simulink model "fm_maja"  (R2025b)
settings: Solver=ode2  StartTime=0.0  StopTime=5  FixedStep=vehicle.sampletime  RelTol=1e-3  EnableMultiTasking=on
undefined symbols (not defined in the file or in its folder): battery, constants, Earth, engine, F, Light, MIL, propeller, servo, vehicle, WGS84
libraries: sharedtransform x3, aerolibwind2 x2, aerolibutil x2, aerolib6dof2 x1, aerolibatmos2 x1, aerolibtransform2 x1, simulink x1, aerolibobsolete x1
settings Model: Creator=ac112430  LastModifiedBy=ac124458
settings SolverCC: AlgebraicLoopSolver=TrustRegion
settings DataIOCC: ReturnWorkspaceOutputs=off
settings OptimizationCC: ReuseModelBlockBuffer=off  LifeSpan=inf
settings DebuggingCC: UnconnectedInputMsg=warning  UnconnectedOutputMsg=warning  UnconnectedLineMsg=warning  SFUnexpectedBacktrackingDiag=warning  SFNoUnconditionalDefaultTransitionDiag=warning  SFExecutionAtInitializationDiag=none  ArithmeticOperatorsInVariantConditions=warning
settings ModelReferenceCC: EnableRefExpFcnMdlSchedulingChecks=on
settings SFSimCC: SimUseLocalCustomCode=off  CustomCodeUndefinedFunction=UseInterfaceOnly
settings RTWCC: RTWUseLocalCustomCode=off  GPUComputeCapability=3.5
settings CodeAppCC: StateflowObjectComments=on
settings GRTTargetCC: TargetLangStandard=C89/C90 (ANSI)
settings ConfigComp: CovMetricSettings=dw  CovSaveCumulativeToWorkspaceVar=on  CovSaveSingleToWorkspaceVar=on  CovExternalEMLEnable=off

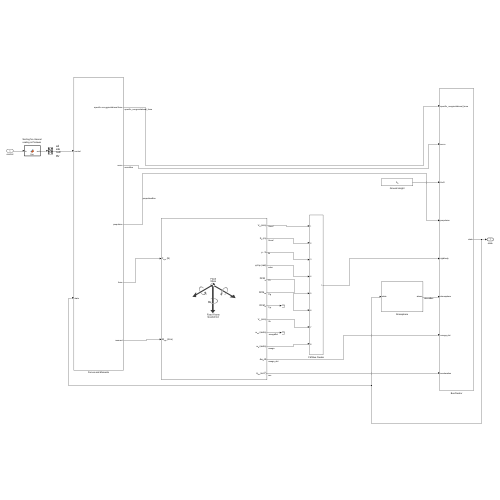
[thumbnail: Simulink's stored preview of the top-level diagram]
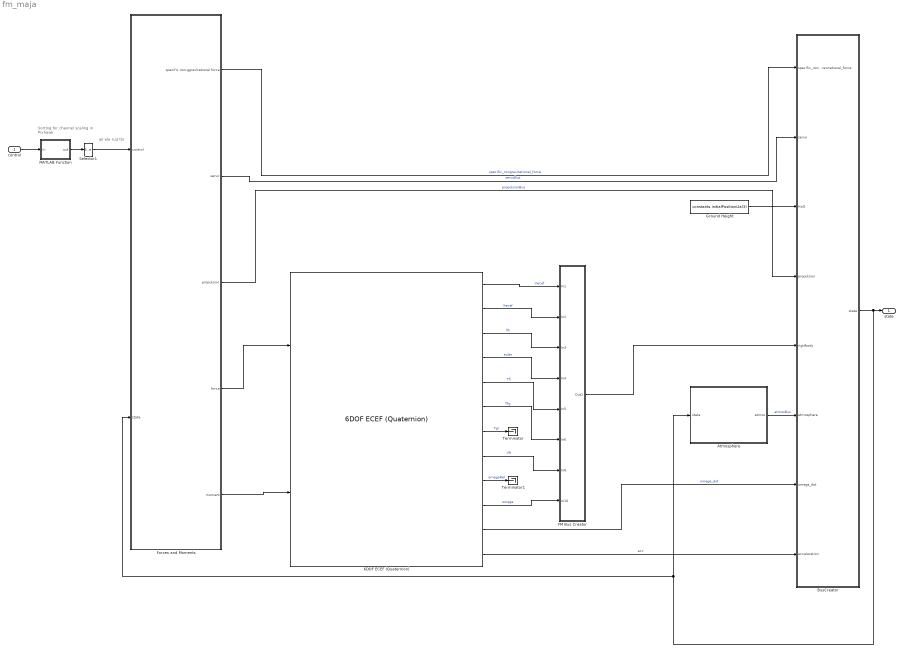
== system fm_maja ==
  note: ail
      | ele
      | rud
      | thr
  note: Sorting for channel
      | scaling in Pixhawk
  control : Inport  PortDimensions=4
  6DOF ECEF (Quaternion) : aerolib6dof2/6DOF ECEF (Quaternion)  units=Metric (MKS)  mtype=Fixed  xg_0=vehicle.pos0  Vm_0=vehicle.v0  eul_0=vehicle.ori0  pm_0=vehicle.omega0  mass_0=vehicle.m  mass_e=0.5  mass_f=2.0  inertia=vehicle.J  inertia_e=eye(3)  inertia_f=2*eye(3)  vre_flag=on  abi_flag=off  ptype=Earth (WGS84)  R=6378137  F=1/298.257223563  w_E=7292115e-11  angle_in=Internal  LPM0=0  quat_statename=''  pm_statename=''  Vm_statename=''  posfixedframe_statename=''  posinertial_statename=''  LPM_statename=''  mass_statename=''
  Atmosphere : Subsystem
  BusCreator : Subsystem
  FM Bus Creator : Subsystem
  Forces and Moments : Subsystem
  Ground Height : Constant  Value=constants.initialPositionLla(3)  SampleTime=-1
      mask Display: disp('h_0', 'texmode', 'on');
  MATLAB Function : MATLAB Function  TreatAsAtomicUnit=on
  Selector1 : Selector  InputPortWidth=4  IndexOptions=Index vector (dialog)  Indices=[2 3 4 1]  OutputSizes=1  RuntimeRangeChecks=on
  Terminator : Terminator
  Terminator1 : Terminator
  state : Outport  OutDataTypeStr=Bus: fmBus  VectorParamsAs1DForOutWhenUnconnected=off
  wires:
  6DOF ECEF (Quaternion)/11 -> BusCreator/7(omega_dot)  "omega_dot"
  BusCreator/1(state) -> Atmosphere/1(state), Forces and Moments/2(state), state/1
  Atmosphere/1(atmos) -> BusCreator/6(atmosphere)  "atmosBus"
  Forces and Moments/1(specific non-ggravitational force) -> BusCreator/1(specific_nongravitational_force)  "specific_nongravitational_force"
  Forces and Moments/2(servo) -> BusCreator/2(servo)  "servoBus"
  Forces and Moments/3(propulsion) -> BusCreator/4(propulsion)  "propulsionBus"
  Forces and Moments/5(moment) -> 6DOF ECEF (Quaternion)/2
  Forces and Moments/4(force) -> 6DOF ECEF (Quaternion)/1
  control/1 -> MATLAB Function/1(in)
  Ground Height/1 -> BusCreator/3(HoG)
  6DOF ECEF (Quaternion)/12 -> BusCreator/8(acceleration)  "acc"
  6DOF ECEF (Quaternion)/1 -> FM Bus Creator/1(In1)  "Vecef"
  6DOF ECEF (Quaternion)/2 -> FM Bus Creator/2(In2)  "Xecef"
  6DOF ECEF (Quaternion)/3 -> FM Bus Creator/3(In3)  "llh"
  6DOF ECEF (Quaternion)/4 -> FM Bus Creator/4(In4)  "euler"
  6DOF ECEF (Quaternion)/5 -> FM Bus Creator/5(In5)  "Tfi"
  6DOF ECEF (Quaternion)/6 -> FM Bus Creator/6(In6)  "Tfg"
  6DOF ECEF (Quaternion)/8 -> FM Bus Creator/7(In8)  "Vb"
  6DOF ECEF (Quaternion)/10 -> FM Bus Creator/8(In10)  "omega"
  FM Bus Creator/1(Out1) -> BusCreator/5(rigidbody)
  6DOF ECEF (Quaternion)/9 -> Terminator1/1  "omegaRel"
  6DOF ECEF (Quaternion)/7 -> Terminator/1  "Tgr"
  MATLAB Function/1(out) -> Selector1/1
  Selector1/1 -> Forces and Moments/1(control)

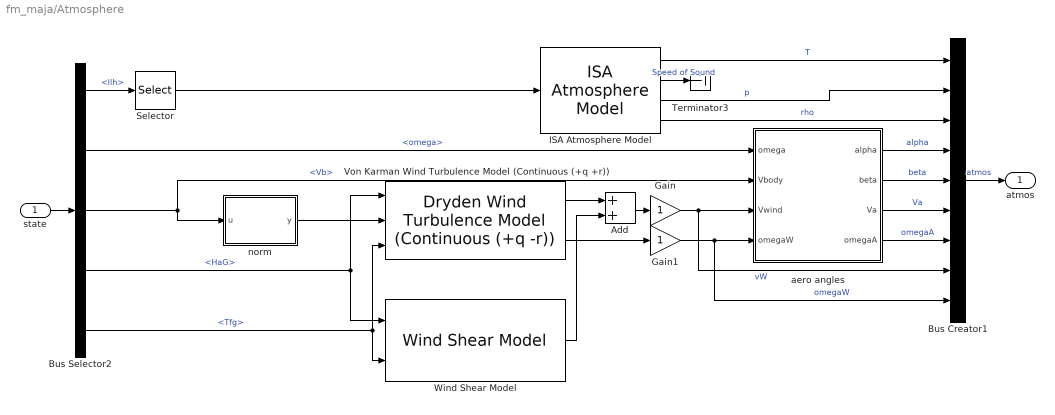
== system fm_maja/Atmosphere ==
  state : Inport
  Add : Sum
  Bus Creator1 : BusCreator  Inputs=9  OutDataTypeStr=Bus: atmosBus
  Bus Selector2 : BusSelector  OutputSignals=rigidbodyBus.llh,rigidbodyBus.omega,rigidbodyBus.Vb,utilityBus.HaG,rigidbodyBus.Tfg
  Gain : Gain
  Gain1 : Gain
  ISA Atmosphere Model : aerolibatmos2/ISA Atmosphere Model  useExtended=off  action=Warning  custom=off  viscosityOut=off  g=9.80665  gamma=1.4  R=287.0531  L=0.0065  h_trop=11000  h_strat=20000  rho0=1.225  P0=101325  T0=288.15  h0=0  S=110.4  Tref=273.15  muref=1.716e-5
  Selector : Selector  InputPortWidth=3  IndexOptions=Index vector (dialog)  Indices=3  OutputSizes=1
  Terminator3 : Terminator
  Von Karman Wind Turbulence Model (Continuous (+q +r)) : aerolibwind2/Dryden Wind Turbulence Model  (Continuous (+q -r))  units=Metric (MKS)  spec=MIL-F-8785C  model=Continuous Von Karman (+q +r)  W20=atmosphere.windStrength  Wdeg=atmosphere.windDir  TurbProb=10^-2 - Light  L_high=410  Wingspan=aerodynamic.b  ts=vehicle.sampletime  Seed=randi(20000,1,4)  T_on=off
  Wind Shear Model : aerolibwind2/Wind Shear Model  units=Metric (MKS)  phase=Other  W_20=atmosphere.windStrength  Wdeg=atmosphere.windDir
  aero angles : MATLAB Function  TreatAsAtomicUnit=on
  norm : MATLAB Function  TreatAsAtomicUnit=on
  atmos : Outport  VectorParamsAs1DForOutWhenUnconnected=off
  wires:
  Bus Creator1/1 -> atmos/1  "atmos"
  ISA Atmosphere Model/3 -> Bus Creator1/2  "p"
  ISA Atmosphere Model/1 -> Bus Creator1/1  "T"
  ISA Atmosphere Model/2 -> Terminator3/1  "Speed of Sound"
  Bus Selector2/1 -> Selector/1  "<llh>"
  Selector/1 -> ISA Atmosphere Model/1
  ISA Atmosphere Model/4 -> Bus Creator1/3  "rho"
  aero angles/3(Va) -> Bus Creator1/6  "Va"
  aero angles/1(alpha) -> Bus Creator1/4  "alpha"
  aero angles/2(beta) -> Bus Creator1/5  "beta"
  state/1 -> Bus Selector2/1
  Bus Selector2/2 -> aero angles/1(omega)  "<omega>"
  Bus Selector2/3 -> aero angles/2(Vbody), norm/1(u)  "<Vb>"
  Wind Shear Model/1 -> Add/2
  norm/1(y) -> Von Karman Wind Turbulence Model (Continuous (+q +r))/2
  Von Karman Wind Turbulence Model (Continuous (+q +r))/1 -> Add/1
  Von Karman Wind Turbulence Model (Continuous (+q +r))/2 -> Gain1/1
  Add/1 -> Gain/1
  Bus Selector2/5 -> Wind Shear Model/2, Von Karman Wind Turbulence Model (Continuous (+q +r))/3  "<Tfg>"
  aero angles/4(omegaA) -> Bus Creator1/7  "omegaA"
  Bus Selector2/4 -> Wind Shear Model/1, Von Karman Wind Turbulence Model (Continuous (+q +r))/1  "<HaG>"
  Gain/1 -> Bus Creator1/8, aero angles/3(Vwind)  "vW"
  Gain1/1 -> Bus Creator1/9, aero angles/4(omegaW)  "omegaW"

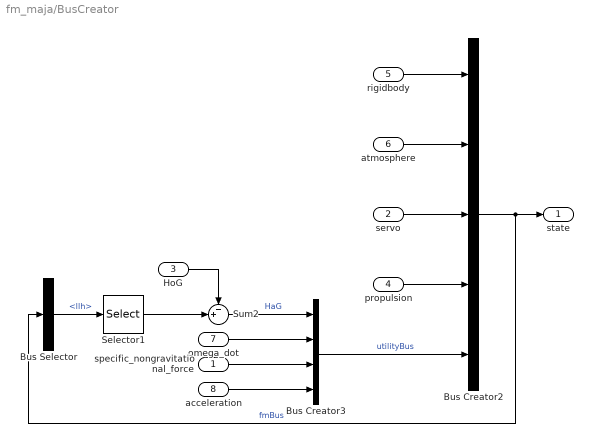
== system fm_maja/BusCreator ==
  specific_nongravitational_force : Inport
  servo : Inport  Port=2
  HoG : Inport  Port=3
  propulsion : Inport  Port=4
  rigidbody : Inport  Port=5
  atmosphere : Inport  Port=6
  omega_dot : Inport  Port=7
  acceleration : Inport  Port=8
  Bus Creator2 : BusCreator  Inputs=5
  Bus Creator3 : BusCreator  Inputs=4  OutDataTypeStr=Bus: utilityBus
  Bus Selector : BusSelector  OutputSignals=rigidbodyBus.llh
  Selector1 : Selector  InputPortWidth=3  IndexOptions=Index vector (dialog)  Indices=3  OutputSizes=1
  Sum2 : Sum  Inputs=-+|
  state : Outport  VectorParamsAs1DForOutWhenUnconnected=off
  wires:
  Sum2/1 -> Bus Creator3/1  "HaG"
  propulsion/1 -> Bus Creator2/4
  servo/1 -> Bus Creator2/3
  Bus Creator3/1 -> Bus Creator2/5  "utilityBus"
  Bus Creator2/1 -> state/1, Bus Selector/1  "fmBus"
  atmosphere/1 -> Bus Creator2/2
  Bus Selector/1 -> Selector1/1  "<llh>"
  rigidbody/1 -> Bus Creator2/1
  specific_nongravitational_force/1 -> Bus Creator3/3
  Selector1/1 -> Sum2/2
  HoG/1 -> Sum2/1
  omega_dot/1 -> Bus Creator3/2
  acceleration/1 -> Bus Creator3/4

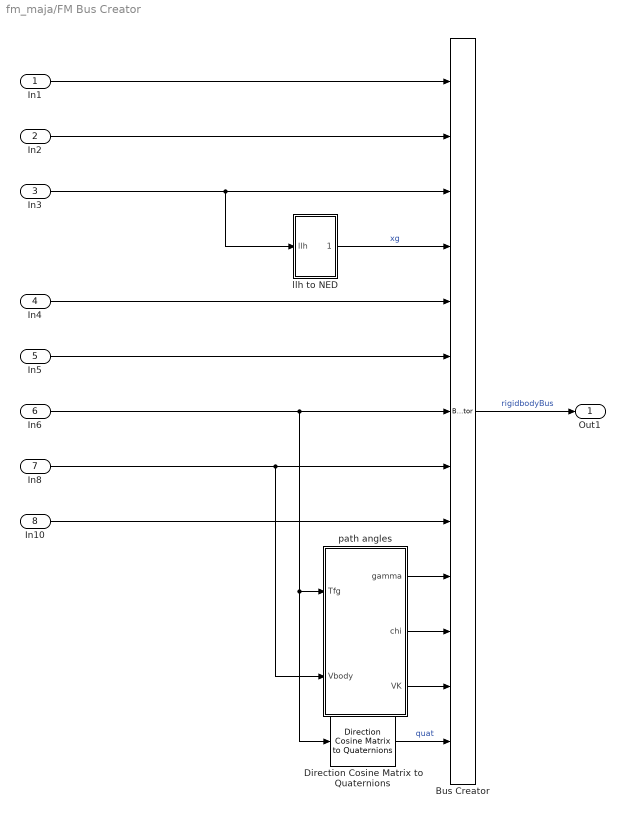
== system fm_maja/FM Bus Creator ==
  In1 : Inport
  In2 : Inport  Port=2
  In3 : Inport  Port=3
  In4 : Inport  Port=4
  In5 : Inport  Port=5
  In6 : Inport  Port=6
  In8 : Inport  Port=7
  In10 : Inport  Port=8
  Bus Creator : BusCreator  Inputs=13  OutDataTypeStr=Bus: rigidbodyBus
  Direction Cosine Matrix to Quaternions : sharedtransform/Direction Cosine Matrix  to Quaternions  aMode=aMode  action=None  tolerance=eps(2)
  llh to NED : Subsystem
  path angles : MATLAB Function  TreatAsAtomicUnit=on
  Out1 : Outport  VectorParamsAs1DForOutWhenUnconnected=off
  wires:
  In10/1 -> Bus Creator/9
  path angles/2(chi) -> Bus Creator/11
  path angles/1(gamma) -> Bus Creator/10
  Direction Cosine Matrix to Quaternions/1 -> Bus Creator/13  "quat"
  In1/1 -> Bus Creator/1
  path angles/3(VK) -> Bus Creator/12
  In3/1 -> llh to NED/1(llh), Bus Creator/3
  In2/1 -> Bus Creator/2
  Bus Creator/1 -> Out1/1  "rigidbodyBus"
  In4/1 -> Bus Creator/5
  In8/1 -> path angles/2(Vbody), Bus Creator/8
  In6/1 -> Bus Creator/7, Direction Cosine Matrix to Quaternions/1, path angles/1(Tfg)
  In5/1 -> Bus Creator/6
  llh to NED/1(NED) -> Bus Creator/4  "xg"

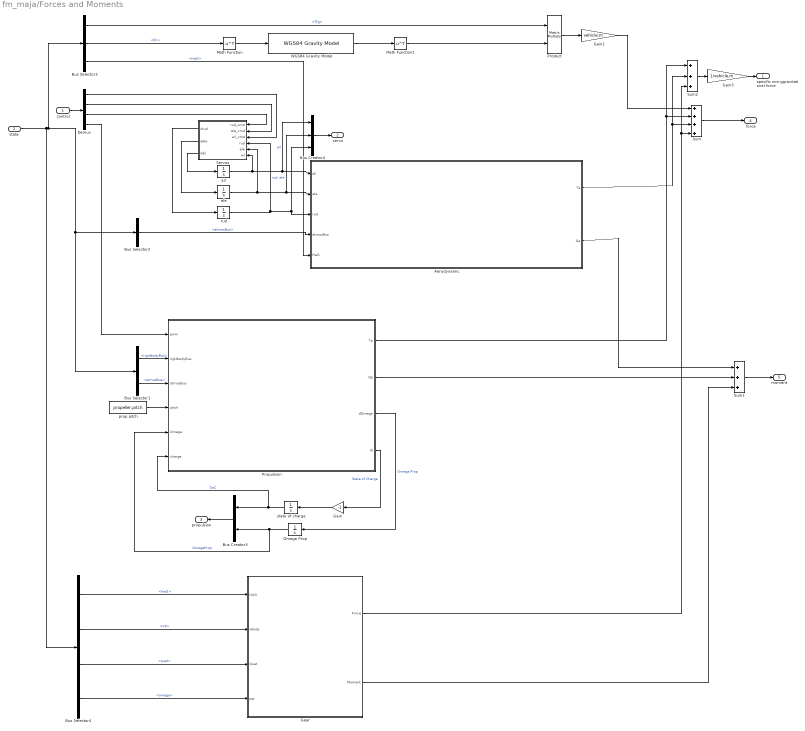
== system fm_maja/Forces and Moments ==
  control : Inport
  state : Inport  Port=2
  Aerodynamic : MATLAB Function  TreatAsAtomicUnit=on
  Bus Creator3 : BusCreator  Inputs=2  OutDataTypeStr=Bus: propulsionBus
  Bus Creator4 : BusCreator  Inputs=3  OutDataTypeStr=Bus: servoBus
  Bus Selector1 : BusSelector  OutputSignals=rigidbodyBus,atmosBus
  Bus Selector2 : BusSelector  OutputSignals=atmosBus
  Bus Selector3 : BusSelector  OutputSignals=rigidbodyBus.Tfg,rigidbodyBus.llh,utilityBus.HaG
  Bus Selector4 : BusSelector  OutputSignals=utilityBus.HaG,rigidbodyBus.Vb,rigidbodyBus.quat,rigidbodyBus.omega
  Demux : Demux
  Gain : Gain  Gain=-1
  Gain1 : Gain  Gain=vehicle.m
  Gain3 : Gain  Gain=1/vehicle.m
  Gear : Subsystem
  Math Function : Math  Operator=transpose  SignedPower=on
  Math Function1 : Math  Operator=transpose  SignedPower=on
  Omega Prop : Integrator  InitialCondition=engine.Omega0
  Product : Product  Multiplication=Matrix(*)
  Propulsion : MATLAB Function  TreatAsAtomicUnit=on
  Servos : MATLAB Function  TreatAsAtomicUnit=on
  Sum : Sum  Inputs=++++
  Sum1 : Sum  Inputs=+++
  Sum2 : Sum  Inputs=+++
  "WGS84 Gravity Model " : aerolibobsolete/WGS84 Gravity Model   model=WGS84 Taylor Series  units=Metric (MKS)  no_atmos=on  precessing=on  jd_loc=off  month=October  day=10  year=2004  no_centrifugal=on  action=Warning
  ail : Integrator  LimitOutput=on  UpperSaturationLimit=servo.ailLim(1)  LowerSaturationLimit=servo.ailLim(2)
  ele : Integrator  LimitOutput=on  UpperSaturationLimit=servo.eleLim(1)  LowerSaturationLimit=servo.eleLim(2)
  prop pitch : Constant  Value=propeller.pitch
  rud : Integrator  LimitOutput=on  UpperSaturationLimit=servo.rudLim(1)  LowerSaturationLimit=servo.rudLim(2)
  state of charge : Integrator  InitialCondition=battery.Qnom
  specific non-ggravitational force : Outport  VectorParamsAs1DForOutWhenUnconnected=off
  servo : Outport  Port=2  VectorParamsAs1DForOutWhenUnconnected=off
  propulsion : Outport  Port=3  VectorParamsAs1DForOutWhenUnconnected=off
  force : Outport  Port=4  VectorParamsAs1DForOutWhenUnconnected=off
  moment : Outport  Port=5  VectorParamsAs1DForOutWhenUnconnected=off
  wires:
  Propulsion/3(dOmega) -> Omega Prop/1  "Omega Prop"
  Omega Prop/1 -> Bus Creator3/2, Propulsion/5(Omega)  "OmegaProp"
  prop pitch/1 -> Propulsion/4(pitch)
  Math Function/1 -> "WGS84 Gravity Model "/1
  Propulsion/4(Ib) -> Gain/1  "State of Charge"
  Gain/1 -> state of charge/1
  "WGS84 Gravity Model "/1 -> Math Function1/1
  Math Function1/1 -> Product/2
  Product/1 -> Gain1/1
  Bus Creator3/1 -> propulsion/1
  Propulsion/1(Tp) -> Sum2/1, Sum/2
  Gain1/1 -> Sum/1
  state of charge/1 -> Propulsion/6(charge), Bus Creator3/1  "SoC"
  Servos/2(dele) -> ele/1
  Sum1/1 -> moment/1
  ele/1 -> Servos/5(ele), Bus Creator4/2, Aerodynamic/2(ele)  "ele"
  rud/1 -> Servos/4(rud), Bus Creator4/3, Aerodynamic/3(rud)  "rud"
  Sum/1 -> force/1
  ail/1 -> Bus Creator4/1, Aerodynamic/1(ail), Servos/6(ail)  "ail"
  Servos/3(dail) -> ail/1
  Servos/1(drud) -> rud/1
  Demux/2 -> Servos/2(ele_cmd)
  Demux/1 -> Servos/3(ail_cmd)
  Demux/3 -> Servos/1(rud_cmd)
  control/1 -> Demux/1
  Bus Creator4/1 -> servo/1
  Bus Selector4/2 -> Gear/2(vBody)  "<Vb>"
  Bus Selector4/4 -> Gear/4(pqr)  "<omega>"
  Demux/4 -> Propulsion/1(pwm)
  Bus Selector4/3 -> Gear/3(Quat)  "<quat>"
  Aerodynamic/1(Ta) -> Sum2/2, Sum/3
  Sum2/1 -> Gain3/1
  Gain3/1 -> specific non-ggravitational force/1
  Aerodynamic/2(Qa) -> Sum1/1
  Propulsion/2(Qp) -> Sum1/2
  Bus Selector1/1 -> Propulsion/2(rigidbodyBus)  "<rigidbodyBus>"
  Bus Selector1/2 -> Propulsion/3(atmosBus)  "<atmosBus>"
  Bus Selector2/1 -> Aerodynamic/4(atmosBus)  "<atmosBus>"
  Gear/1(Force) -> Sum2/3, Sum/4
  Gear/2(Moment) -> Sum1/3
  Bus Selector4/1 -> Gear/1(HAG)  "<HaG>"
  Bus Selector3/1 -> Product/1  "<Tfg>"
  Bus Selector3/2 -> Math Function/1  "<llh>"
  Bus Selector3/3 -> Aerodynamic/5(HaG)  "<HaG>"
  state/1 -> Bus Selector2/1, Bus Selector1/1, Bus Selector3/1, Bus Selector4/1

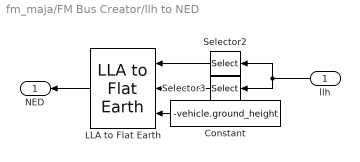
== system fm_maja/FM Bus Creator/llh to NED ==
  llh : Inport
  Constant : Constant  Value=-vehicle.ground_height
  LLA to Flat Earth : aerolibtransform2/LLA to Flat Earth  units=Metric (MKS)  ptype=Earth (WGS84)  F=1/298.257223563  R=6378137  refPosPort=off  LL0=vehicle.pos0(1:2)  psi=0
  Selector2 : Selector  InputPortWidth=3  IndexOptions=Index vector (dialog)  Indices=1:2  OutputSizes=1
  Selector3 : Selector  InputPortWidth=3  IndexOptions=Index vector (dialog)  Indices=3  OutputSizes=1
  NED : Outport  VectorParamsAs1DForOutWhenUnconnected=off
  wires:
  LLA to Flat Earth/1 -> NED/1
  llh/1 -> Selector3/1, Selector2/1
  Constant/1 -> LLA to Flat Earth/3
  Selector2/1 -> LLA to Flat Earth/1
  Selector3/1 -> LLA to Flat Earth/2

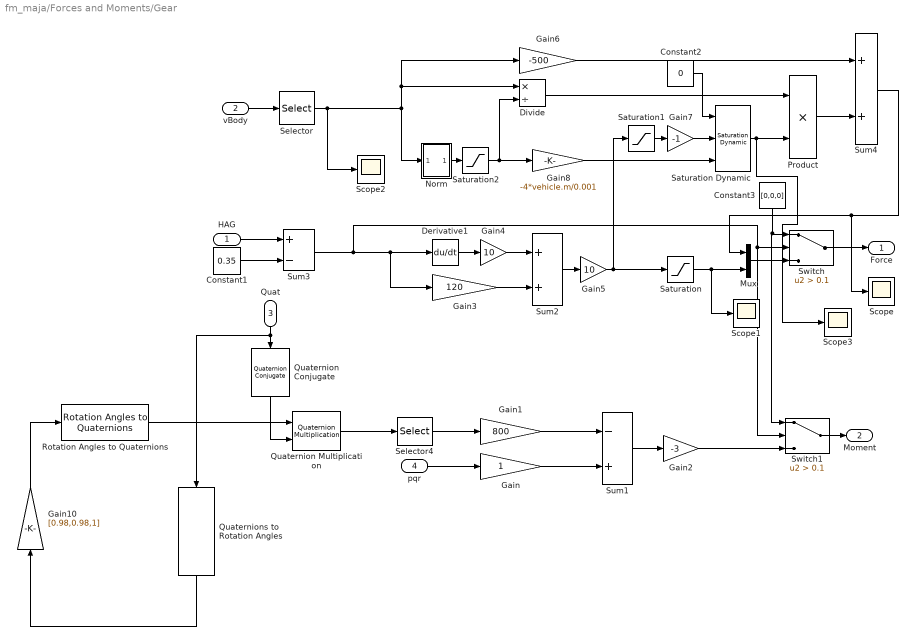
== system fm_maja/Forces and Moments/Gear ==
  HAG : Inport
  vBody : Inport  Port=2
  Quat : Inport  Port=3
  pqr : Inport  Port=4
  Constant1 : Constant  Value=0.35  SampleTime=-1
  Constant2 : Constant  Value=0  SampleTime=-1
  Constant3 : Constant  Value=[0,0,0]  SampleTime=-1
  Derivative1 : Derivative  CoefficientInTFapproximation=5
  Divide : Product  Inputs=*/
  Gain : Gain
  Gain1 : Gain  Gain=800
  Gain10 : Gain  Gain=[0.98,0.98,1]
  Gain2 : Gain  Gain=-3
  Gain3 : Gain  Gain=120
  Gain4 : Gain  Gain=10
  Gain5 : Gain  Gain=10
  Gain6 : Gain  Gain=-500
  Gain7 : Gain  Gain=-1
  Gain8 : Gain  Gain=-4*vehicle.m/0.001
  Mux : Mux  Inputs=2
  Norm : Subsystem
  Product : Product
  Quaternion Conjugate : aerolibutil/Quaternion Conjugate
  Quaternion Multiplication : aerolibutil/Quaternion Multiplication
  Quaternions to Rotation Angles : sharedtransform/Quaternions to Rotation Angles  rotationOrder=XYZ  aMode=aMode
  Rotation Angles to Quaternions : sharedtransform/Rotation Angles to Quaternions  rotationOrder=XYZ  aMode=aMode
  Saturation : Saturate  UpperLimit=800  LowerLimit=-800
  Saturation Dynamic : simulink/Discontinuities/Saturation Dynamic  OutMin=[]  OutMax=[]  OutDataTypeStr=Inherit: Same as second input  OutDataType=fixdt(1, 16)  OutScaling=2^-10  DoSatur=off
  Saturation1 : Saturate  UpperLimit=0  LowerLimit=-20
  Saturation2 : Saturate  UpperLimit=100  LowerLimit=0.01
  Scope{,1..3} (4 alike) : Scope
      Scope settings: ActiveDisplayYMinimum=-1145.67531  ActiveDisplayYMaximum=137.03268
      Scope1 settings: ActiveDisplayYMinimum=-501.58961  ActiveDisplayYMaximum=944.62107
      Scope2 settings: ActiveDisplayYMinimum=-2.74065  ActiveDisplayYMaximum=22.91351  DataLoggingVariableName=ScopeData4
      Scope3 settings: ActiveDisplayYMinimum=-1  ActiveDisplayYMaximum=1  DataLoggingVariableName=ScopeData5
  Selector : Selector  InputPortWidth=3  IndexOptions=Index vector (dialog)  Indices=1:2  OutputSizes=1
  Selector4 : Selector  InputPortWidth=4  IndexOptions=Index vector (dialog)  Indices=2:4  OutputSizes=1
  Sum1 : Sum  Inputs=-+
  Sum2 : Sum
  Sum3 : Sum  Inputs=+-
  Sum4 : Sum
  Switch : Switch  Criteria=u2 > Threshold  Threshold=0.1  SaturateOnIntegerOverflow=off  InputSameDT=off
  Switch1 : Switch  Criteria=u2 > Threshold  Threshold=0.1  SaturateOnIntegerOverflow=off  InputSameDT=off
  Force : Outport  VectorParamsAs1DForOutWhenUnconnected=off
  Moment : Outport  Port=2  VectorParamsAs1DForOutWhenUnconnected=off
  wires:
  Gain3/1 -> Sum2/2
  pqr/1 -> Gain/1
  Gain1/1 -> Sum1/1
  Derivative1/1 -> Gain4/1
  Sum2/1 -> Gain5/1
  Sum1/1 -> Gain2/1
  Gain4/1 -> Sum2/1
  vBody/1 -> Selector/1
  Quat/1 -> Quaternions to Rotation Angles/1, Quaternion Conjugate/1
  Constant1/1 -> Sum3/2
  Gain5/1 -> Saturation/1, Saturation1/1
  Saturation/1 -> Scope1/1, Mux/2
  Mux/1 -> Switch/3
  Switch/1 -> Force/1
  HAG/1 -> Sum3/1
  Constant3/1 -> Switch1/1, Switch/1
  Saturation1/1 -> Gain7/1
  Gain7/1 -> Saturation Dynamic/2
  Saturation Dynamic/1 -> Scope3/1, Product/2
  Constant2/1 -> Saturation Dynamic/1
  Gain8/1 -> Saturation Dynamic/3
  Switch1/1 -> Moment/1
  Norm/1(Out1) -> Saturation2/1
  Divide/1 -> Product/1
  Saturation2/1 -> Divide/2, Gain8/1
  Sum4/1 -> Scope/1, Mux/1
  Gain6/1 -> Sum4/1
  Quaternion Multiplication/1 -> Selector4/1
  Gain2/1 -> Switch1/3
  Sum3/1 -> Switch1/2, Switch/2, Gain3/1, Derivative1/1
  Gain/1 -> Sum1/2
  Quaternions to Rotation Angles/1 -> Gain10/1
  Gain10/1 -> Rotation Angles to Quaternions/1
  Selector4/1 -> Gain1/1
  Quaternion Conjugate/1 -> Quaternion Multiplication/2
  Rotation Angles to Quaternions/1 -> Quaternion Multiplication/1
  Selector/1 -> Scope2/1, Gain6/1, Divide/1, Norm/1(In1)
  Product/1 -> Sum4/2

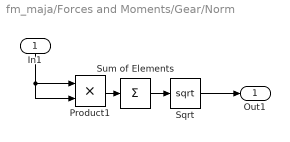
== system fm_maja/Forces and Moments/Gear/Norm ==
  In1 : Inport
  Product1 : Product
  Sqrt : Sqrt
  Sum of Elements : Sum  Inputs=+
  Out1 : Outport  VectorParamsAs1DForOutWhenUnconnected=off
  wires:
  In1/1 -> Product1/2, Product1/1
  Sum of Elements/1 -> Sqrt/1
  Product1/1 -> Sum of Elements/1
  Sqrt/1 -> Out1/1

== matlab function fm_maja/Atmosphere/norm ==
  data: u input; y output
function y = norm(u)
%#codegen

y = norm(u);
if y < 1
    y = 1;
end

== matlab function fm_maja/MATLAB Function ==
  data: in input; out output
function out = fcn(in)
out = zeros(4,1);

out(1) = in(1); %thr
out(2) = in(2); %ail
out(3) = 1/sqrt(2)*(in(6)+in(7)); %ele
out(4) = 1/sqrt(2)*(in(6)-in(7)); %rud

== matlab function fm_maja/Atmosphere/aero angles ==
  data: omega input size=3; Vbody input; Vwind input; omegaW input size=3; alpha output; beta output; Va output; omegaA output size=3
function [alpha,beta,Va,omegaA] = calcAeroAngles(omega,Vbody,Vwind,omegaW)
bVa = Vbody+Vwind;
if abs(bVa(1))>1
    alpha = atan2(bVa(3),bVa(1));
else
    alpha = 0;
end
if norm(bVa)>1
    beta  = asin(bVa(2)/norm(bVa));
else
    beta = 0;
end
Va    = norm(bVa);
omegaA = omega + omegaW;

== matlab function fm_maja/Forces and Moments/Propulsion ==
  data: pwm input; Tp output; rigidbodyBus input; atmosBus input; Qp output; pitch input; Omega input; charge input; dOmega output; Ib output; battery parameter; propeller parameter; engine parameter
function [Tp,Qp,dOmega,Ib] = propulsion(pwm,rigidbodyBus,atmosBus,pitch,Omega,charge,battery,propeller,engine)

omega = rigidbodyBus.omega;
Va    = atmosBus.Va;
rho   = atmosBus.rho;

charge = battery.Qnom; % to turn off battery simulation

% deduced propeller properties
aspectRatio = 2*propeller.radius/propeller.chord;
dca = 2*pi*aspectRatio/(2+aspectRatio); % valid for elliptical lift distribution and aspect ratio > 3; cf.Prandtl, Tragflügeltheorie I.
sigma = propeller.blades*propeller.chord/(pi*propeller.radius);
tiploss = 1-propeller.chord/(2*propeller.radius);

% induced velocity
% 	Both the equations and notation in this block is adopted from Johnson, Helicopter Theory(p. 52ff).
% 	Note that the following assumptions are made :
% 	1. Ideally twisted proeller with constant chord
% 	2. Uniform inflow
% 	3. propeller vortex wake interaction neglected
% 	4. Positive inflow ratio (. no thrust reversal)

if abs(Omega) > 0.1*pi
    lambda_c = Va/(Omega*propeller.radius);
    lambda = sqrt((sigma*dca/16-lambda_c/2)^2+sigma*dca*pitch/8)-(sigma*dca/16-lambda_c/2); % combined blade element and momentum theory; Johnson, Helicopter Theory (p. 56f)
    
    % propeller thrust
    thrustCoefficient = sigma*dca/4*(pitch-lambda)*tiploss^2;
    thrust = thrustCoefficient*rho*pi*propeller.radius^2*(propeller.radius^2*Omega*abs(Omega));
    
    % propeller torque;
    inducedDragTorqueCoefficient = thrustCoefficient*lambda;
    airfoilDragTorqueCoefficient = sigma*(propeller.delta(1)/8+((propeller.delta(2)/6)*(pitch-lambda))+((propeller.delta(3)/4)*(pitch-lambda)^2));
    torqueCoefficient = inducedDragTorqueCoefficient+airfoilDragTorqueCoefficient;
    Qa = torqueCoefficient*rho*pi*propeller.radius^3*(propeller.radius^2*Omega*abs(Omega));
else
    thrust = 0;
    Qa = 0;
end

% Olivier Tremblay,A Generic Battery Model for the Dynamic Simulation of Hybrid Electric Vehicles
V0 = battery.Vfull-battery.A;
Ubat = V0+battery.K*(battery.Qfull-charge)/charge+battery.A*exp(-battery.B*(battery.Qfull-charge));

% Isermann Mechatronic Systems
pwm = pwm*0.5+0.5;
pwm = max(0,min(1,pwm));
Ib = (Ubat*pwm-engine.ke*Omega)/(engine.R+battery.R);
if Ib > engine.Imax
    Ib = engine.Imax;
end
Qf = engine.eff*engine.kf*Omega;
if Ib < 0
    Ib = 0;
    Qe = 0;
    dOmega = -Qf/(engine.J+propeller.J);
else
    Qe = engine.ke*Ib;
    dOmega = (Qe-(Qa+Qf))/(engine.J+propeller.J);
end

% Thrust Direction
n = [cos(propeller.if);0;-sin(propeller.if)];
% Thrust vector
Tp = n*thrust;
% Angular Momentum
Lp = n*(engine.J+propeller.J)*Omega;
% Prop torque vector
Qp = -n*(Qe-Qf) + cross(propeller.pos,Tp) - cross(omega,Lp);

end

== matlab function fm_maja/Forces and Moments/Aerodynamic ==
  data: ail input; ele input; rud input; Ta output; atmosBus input; Qa output; aerodynamic parameter; HaG input
function [Ta,Qa] = aerodynamic(ail,ele,rud,atmosBus,aerodynamic,HaG)

omegaA = atmosBus.omegaA;
Va    = atmosBus.Va;
rho   = atmosBus.rho;
alpha = atmosBus.alpha;
beta  = atmosBus.beta;

Tfs = stabilityToBody(alpha);
pdyn = 0.5*rho*Va^2;

if Va > 1
    pstar = omegaA(1)*aerodynamic.b/(2*Va);
    qstar = omegaA(2)*aerodynamic.chord/(2*Va);
    rstar = omegaA(3)*aerodynamic.b/(2*Va);
else
    Valim = 1;
    pstar = omegaA(1)*aerodynamic.b/(2*Valim);
    qstar = omegaA(2)*aerodynamic.chord/(2*Valim);
    rstar = omegaA(3)*aerodynamic.b/(2*Valim);
end

VaLim = lim(Va,aerodynamic.derivatives.vBounds);

% Pitch Rate
CDq  = interp1(aerodynamic.derivatives.VInf,aerodynamic.derivatives.CDq,VaLim);
CLq  = interp1(aerodynamic.derivatives.VInf,aerodynamic.derivatives.CLq,VaLim);
Cmq  = interp1(aerodynamic.derivatives.VInf,aerodynamic.derivatives.Cmq,VaLim);

% Roll Rate
CYp  = interp1(aerodynamic.derivatives.VInf,aerodynamic.derivatives.CYp,VaLim);
Clp  = interp1(aerodynamic.derivatives.VInf,aerodynamic.derivatives.Clp,VaLim);
Cnp  = interp1(aerodynamic.derivatives.VInf,aerodynamic.derivatives.Cnp,VaLim);

% Yaw Rate
CYr  = interp1(aerodynamic.derivatives.VInf,aerodynamic.derivatives.CYr,VaLim);
Clr  = interp1(aerodynamic.derivatives.VInf,aerodynamic.derivatives.Clr,VaLim);
Cnr  = interp1(aerodynamic.derivatives.VInf,aerodynamic.derivatives.Cnr,VaLim);

% Elevator
CDele  = interp1(aerodynamic.derivatives.VInf,aerodynamic.derivatives.CDele,VaLim);
CLele  = interp1(aerodynamic.derivatives.VInf,aerodynamic.derivatives.CLele,VaLim);
Cmele  = interp1(aerodynamic.derivatives.VInf,aerodynamic.derivatives.Cmele,VaLim);

% Aileron
CYail  = aerodynamic.derivatives.CYail;
Clail  = aerodynamic.derivatives.Clail;
Cnail  = aerodynamic.derivatives.Cnail;

% Rudder
CYrud  = aerodynamic.derivatives.CYrud;
Clrud  = aerodynamic.derivatives.Clrud;
Cnrud  = aerodynamic.derivatives.Cnrud;


VaLim = lim(Va,aerodynamic.polar.vBounds);
alphaLim = lim(alpha,aerodynamic.polar.alphaBounds);
fbetaLim = lim(abs(beta),aerodynamic.polar.betaBounds);

% Polar
CD = interp3(aerodynamic.polar.beta,aerodynamic.polar.alpha,aerodynamic.polar.V,aerodynamic.polar.CD,fbetaLim,alphaLim,VaLim);
CY = sign(beta)*interp3(aerodynamic.polar.beta,aerodynamic.polar.alpha,aerodynamic.polar.V,aerodynamic.polar.CY,fbetaLim,alphaLim,VaLim);
CL = interp3(aerodynamic.polar.beta,aerodynamic.polar.alpha,aerodynamic.polar.V,aerodynamic.polar.CL,fbetaLim,alphaLim,VaLim);
Cl = sign(beta)*interp3(aerodynamic.polar.beta,aerodynamic.polar.alpha,aerodynamic.polar.V,aerodynamic.polar.Cl,fbetaLim,alphaLim,VaLim);
Cn = sign(beta)*interp3(aerodynamic.polar.beta,aerodynamic.polar.alpha,aerodynamic.polar.V,aerodynamic.polar.Cn,fbetaLim,alphaLim,VaLim);
[alphaGE,CL,CD] = groundEffect(alpha,CL,CD,HaG,aerodynamic.b,aerodynamic.chord,aerodynamic.alpha0); 
alphaLimGE = lim(alphaGE,aerodynamic.polar.alphaBounds);
Cm = interp3(aerodynamic.polar.beta,aerodynamic.polar.alpha,aerodynamic.polar.V,aerodynamic.polar.Cm,fbetaLim,alphaLimGE,VaLim);

% Aggregation
CD = CD + CDq*qstar + CDele*ele;
CL = CL + CLq*qstar + CLele*ele;
CY = CY + CYp*pstar + CYr*rstar + CYail*ail + CYrud*rud;
Cl = Cl + Clp*pstar + Clr*rstar + Clail*ail + Clrud*rud;
Cm = Cm + Cmq*qstar + Cmele*ele;
Cn = Cn + Cnp*pstar + Cnr*rstar + Cnail*ail + Cnrud*rud;


% Force and Torque in wind frame
aTa = [-CD;CY;-CL]*pdyn*aerodynamic.S;
aQa = [Cl*aerodynamic.b;Cm*aerodynamic.chord;Cn*aerodynamic.b]*pdyn*aerodynamic.S;

% Force and Torque in body frame
Ta = Tfs*aTa;
Qa = Tfs*aQa;

end

function [alpha,CL,CD] = groundEffect(alpha,CL,CD,HaG,b,c,alpha0)

%  b: Spannweite, t: Profiltiefe
t       = c/12;  % Profildicke, Schätzung!
e       = 0.8;   % Oswald
AR      = b/c;   % Streckung
CLalpha = liftSlope(AR,0,0); % Endliche ebene Platte, Pfeilung = 0

% Ground Effect Parameters
WaG    = [ 0, 0.1, 0.2, 0.3, 0.4, 0.5, 0.6, 0.7, 0.8, 0.9, 1.0, 1.1, 1.2, 1.3, 1.4, 1.5, 1.6, 1.7, 1.8, 1.9, 2.0];
AACOef = [ 0, 0.3, 0.5, 0.6, 0.68, 0.73, 0.77, 0.82, 0.855, 0.885,0.915, 0.93, 0.94, 0.965, 0.973, 0.98, 0.985, 0.99, 0.995, 1, 1];

Wing_hag = HaG/b;
Cord_hag = HaG/t;

if (Wing_hag < 0.01)
    Wing_hag = 0.01;
end

if (Wing_hag < 2)

    ind = sum(WaG < Wing_hag) + 1;
    
    sigma   = (1 - 1.32*Wing_hag)/(1.05 + 7.4*Wing_hag);
    if sigma < 0
        sigma = 0;
    end
    CD = CD - sigma*(CL^2)/(pi*AR*e); % Calculated with out of GE lift!
    
    AReff      = AR/interp1(WaG,AACOef,Wing_hag);
    CLalphaEff = liftSlope(AReff,0,0);
    dalpha0    = t/c*pi*(3.5655/Cord_hag - 0.1177/Cord_hag^2)/180.0;

    CL = CL-CLalpha*(alpha-alpha0)+CLalphaEff*(alpha - dalpha0 - alpha0);
    alpha = alpha - dalpha0;

end

end

function Cla = liftSlope(AR,lambda,Ma)
    Cla0 = 2*pi; % Auftriebsanstieg Profil
    Cla = Cla0*cos(lambda)/(sqrt(1-Ma^2*cos(lambda)^2+(Cla0*cos(lambda)/(pi*AR))^2)+Cla0*cos(lambda)/(pi*AR));
end

function t = stabilityToBody(alpha)
t = [cos(alpha) 0 -sin(alpha); 0 1 0; sin(alpha) 0 cos(alpha)];
end

function y = lim(y,bounds)
    y = max(bounds(1),min(bounds(2),y));
end

== matlab function fm_maja/FM Bus Creator/path angles ==
  data: Tfg input; Vbody input; gamma output; chi output; VK output
function [gamma,chi,VK] = calcPathAngles(Tfg,Vbody)
VK = Tfg'*Vbody;
if norm(VK)>0.1
    gamma = -asin(VK(3)/norm(VK));
else
    gamma = 0;
end
chi   = atan2(VK(2),VK(1));

== matlab function fm_maja/Forces and Moments/Servos ==
  data: rud_cmd input; ele_cmd input; drud output; dele output; dail output; ail_cmd input; rud input; ele input; ail input; servo parameter
function [drud,dele,dail] = aerodynamic(rud_cmd,ele_cmd,ail_cmd,rud,ele,ail,servo)
dail = 1/servo.T*(ail_cmd*servo.pwmToAngle(1)-ail);
dele = 1/servo.T*(ele_cmd*servo.pwmToAngle(2)-ele);
drud = 1/servo.T*(rud_cmd*servo.pwmToAngle(3)-rud);
end
